simulink model "HVDCMMCInterconnection"  (R2023b)
settings: Solver=FixedStepDiscrete  StartTime=0.0  StopTime=10  FixedStep=Ts_Power  RelTol=1e-4
PreLoadFcn:
  | HVDCMMCInterconnectionParam
StartFcn:
  | tic
StopFcn:
  | toc
values from neighbouring files (symbols this model uses):
  C_PM = 1.758e-3    (= 0.001758)    [HVDCMMCInterconnectionParam.m]
  Cg = 50e-9    (= 5e-08)    [HVDCMMCInterconnectionParam.m]
  D_R = 0.001    [HVDCMMCInterconnectionParam.m]
  D_Rs = 1e8    (= 100000000)    [HVDCMMCInterconnectionParam.m]
  D_Vf = 0    [HVDCMMCInterconnectionParam.m]
  Fnom = 50    [HVDCMMCInterconnectionParam.m]
  HRM = 2    [HVDCMMCInterconnectionParam.m]
  Ki_Ireg = 6    [HVDCMMCInterconnectionParam.m]
  Ki_Preg = 1.0    (= 1)    [HVDCMMCInterconnectionParam.m]
  Ki_Qreg = 1.0    (= 1)    [HVDCMMCInterconnectionParam.m]
  Ki_VDCreg = 100    [HVDCMMCInterconnectionParam.m]
  Kp_Ireg = 0.6    [HVDCMMCInterconnectionParam.m]
  Kp_Preg = 0.5/3    (= 0.166666666667)    [HVDCMMCInterconnectionParam.m]
  Kp_Qreg = 0.5/3    (= 0.166666666667)    [HVDCMMCInterconnectionParam.m]
  Kp_VDCreg = 4    [HVDCMMCInterconnectionParam.m]
  L_cable = 15e-3    (= 0.015)    [HVDCMMCInterconnectionParam.m]
  Larm = Larm_pu*(Zb_ac/(2*pi*Fnom))    [HVDCMMCInterconnectionParam.m]
  Lff = Larm_pu/2    (= 0.075)    [HVDCMMCInterconnectionParam.m]
  Limits_Ireg = [ 2.0  -2.0]    [HVDCMMCInterconnectionParam.m]
  Limits_Preg = [ 1.2, 0.8 ]    [HVDCMMCInterconnectionParam.m]
  Limits_Qreg = [ 0.25, -0.25 ]    [HVDCMMCInterconnectionParam.m]
  Limits_VDCreg = [ 2.0  -2.0]    [HVDCMMCInterconnectionParam.m]
  Lxfo = 0.12    [HVDCMMCInterconnectionParam.m]
  Nb_PM = 36    [HVDCMMCInterconnectionParam.m]
  Pnom = 1000e6    (= 1000000000)    [HVDCMMCInterconnectionParam.m]
  R_cable = 0.5    [HVDCMMCInterconnectionParam.m]
  R_startup = 400    [HVDCMMCInterconnectionParam.m]
  Rarm = Rarm_pu*Zb_ac    [HVDCMMCInterconnectionParam.m]
  Rff = Rarm_pu/2    (= 0.00075)    [HVDCMMCInterconnectionParam.m]
  Rg = 100    [HVDCMMCInterconnectionParam.m]
  Rxfo = 0.003    [HVDCMMCInterconnectionParam.m]
  Slope_Pref = 0.5    [HVDCMMCInterconnectionParam.m]
  Slope_Qref = 0.5    [HVDCMMCInterconnectionParam.m]
  Slope_Vdc_ref = Vnom_dc/5    (= 128000)    [HVDCMMCInterconnectionParam.m]
  Tbrk1_On = 0.1    [HVDCMMCInterconnectionParam.m]
  Tbrk2_On = 1.0    (= 1)    [HVDCMMCInterconnectionParam.m]
  Tdeblock = 1.5    [HVDCMMCInterconnectionParam.m]
  Tfault = 9999    [HVDCMMCInterconnectionParam.m]
  Ton_Converter2 = 4    [HVDCMMCInterconnectionParam.m]
  Ton_PQreg = 4    [HVDCMMCInterconnectionParam.m]
  Ton_VDCreg = 1.5    [HVDCMMCInterconnectionParam.m]
  Ts = Ts_Control    (= 4e-05)    [HVDCMMCInterconnectionParam.m]    (also in power_circ2ss_sps_calc.m = 1e-06)
  Ts_Control = 40e-6    (= 4e-05)    [HVDCMMCInterconnectionParam.m]
  Ts_Power = 20e-6    (= 2e-05)    [HVDCMMCInterconnectionParam.m]
  Vb_ac = sqrt(2/3)*Vnom_sec    [HVDCMMCInterconnectionParam.m]
  Vb_dc = Vnom_dc    (= 640000)    [HVDCMMCInterconnectionParam.m]
  Vc0_PM = 0    [HVDCMMCInterconnectionParam.m]
  Vnom_dc = 640e3    (= 640000)    [HVDCMMCInterconnectionParam.m]
  Vnom_prim = 400e3    (= 400000)    [HVDCMMCInterconnectionParam.m]
  Vnom_sec = 333e3    (= 333000)    [HVDCMMCInterconnectionParam.m]
  w = 2*pi*Fnom    (= 314.159265359)    [HVDCMMCInterconnectionParam.m]
undefined symbols (not defined in the file or in its folder): ACDC, ACDC3, DiscIntNeverNeededParam, gcbh, Pcc, S, sps_AC, sps_rtmsupport
libraries: simulink x61, spsControlledVoltageSourceLib x56, spsCurrentMeasurementLib x56, spsDiodeLib x40, spsSeriesRLCBranchLib x32, spsVoltageMeasurementLib x20, powerlib_extras x9, spsHalfBridgeMMCmodel x8, spsGroundLib x7, spsSecondOrderFilterLib x6, spsabctodq0Lib x6, spsMeanLib x3
(part 3 of 11)

== system HVDCMMCInterconnection/Conv 2 ==
  On : Inport
  Add : Sum
  Bus Selector : BusSelector  OutputSignals=Switch current
  Bus Selector1 : BusSelector  OutputSignals=Switch current
  Constant2 : Constant  Value=Vnom_dc/2  SampleTime=Ts_Power
  Conv2SWn : spsIdealSwitchLib/Ideal Switch  Ron=0.001  Lon=0  IC=0  Rs=1e6  Cs=inf  Measurements=on
  Conv2SWp : spsIdealSwitchLib/Ideal Switch  Ron=0.001  Lon=0  IC=0  Rs=1e6  Cs=inf  Measurements=on
  Conv2VSn : spsControlledVoltageSourceLib/Controlled Voltage Source  Initialize=off  Source_Type=AC  Amplitude=0  Phase=0  Frequency=0  Measurements=None
  Conv2VSp : spsControlledVoltageSourceLib/Controlled Voltage Source  Initialize=off  Source_Type=AC  Amplitude=0  Phase=0  Frequency=0  Measurements=None
  Current Measurement1 : spsCurrentMeasurementLib/Current Measurement  PhasorSimulation=off  OutputType=Complex  PSBequivalent=0
  Current Measurement2 : spsCurrentMeasurementLib/Current Measurement  PhasorSimulation=off  OutputType=Complex  PSBequivalent=0
  Gain : Gain  Gain=0.5
  Gain1 : Gain  Gain=-1
  Ground1 : spsGroundLib/Ground  LConnTagsString=a
  Ground2 : spsGroundLib/Ground  LConnTagsString=a
  Voltage Measurement : spsVoltageMeasurementLib/Voltage Measurement  PhasorSimulation=off  OutputType=Complex  PSBequivalent=0
  Voltage Measurement1 : spsVoltageMeasurementLib/Voltage Measurement  PhasorSimulation=off  OutputType=Complex  PSBequivalent=0
  Voltage Measurement2 : spsVoltageMeasurementLib/Voltage Measurement  PhasorSimulation=off  OutputType=Complex  PSBequivalent=0
  + : PMIOPort  Side=Left
  -- : PMIOPort  Port=2  Side=Left
  tag scope: I_Conv2SWn=global, I_Conv2SWp=global, Idc2=global, Vdc2=global, Vdc2b=global, Vdc2t=global
  wires:
  On/1 -> Conv2SWn/1, Conv2SWp/1
  Current Measurement1/1 -> Add/1
  Current Measurement2/1 -> Gain1/1
  Add/1 -> Gain/1
  Gain/1 -> [Idc2]
  Gain1/1 -> Add/2
  Constant2/1 -> Conv2VSp/1, Conv2VSn/1
  Voltage Measurement/1 -> [Vdc2]
  Voltage Measurement1/1 -> [Vdc2t]
  Voltage Measurement2/1 -> [Vdc2b]
  Conv2SWp/1 -> Bus Selector/1
  Bus Selector/1 -> [I_Conv2SWp]  "<Switch current>"
  Conv2SWn/1 -> Bus Selector1/1
  Bus Selector1/1 -> [I_Conv2SWn]  "<Switch current>"
  connections:
  Conv2SWp/LConn1 -- Current Measurement1/RConn1
  Conv2VSn/LConn1 -- Conv2SWn/RConn1
  Conv2SWp/RConn1 -- Conv2VSp/RConn1
  Conv2VSn/RConn1 -- Conv2VSp/LConn1 -- Ground1/LConn1
  Current Measurement1/LConn1 -- Voltage Measurement/LConn1 -- +/RConn1 -- Voltage Measurement1/LConn1
  --/RConn1 -- Current Measurement2/LConn1 -- Voltage Measurement/LConn2 -- Voltage Measurement2/LConn2
  Current Measurement2/RConn1 -- Conv2SWn/LConn1
  Voltage Measurement1/LConn2 -- Voltage Measurement2/LConn1 -- Ground2/LConn1

== system HVDCMMCInterconnection/DC & converter 2 ==
  Add : Sum
  Cinv : spsSeriesRLCBranchLib/Series RLC Branch  LConnTagsString=__new0  RConnTagsString=__new0  BranchType=RC  Resistance=1e-3  Inductance=1e-3  SetiL0=off  InitialCurrent=0  Capacitance=C_PM/Nb_PM*3  Setx0=off  InitialVoltage=Vnom_dc/2  Measurements=None
  Cinv1 : spsSeriesRLCBranchLib/Series RLC Branch  LConnTagsString=__new0  RConnTagsString=__new0  BranchType=RC  Resistance=1e-3  Inductance=1e-3  SetiL0=off  InitialCurrent=0  Capacitance=C_PM/Nb_PM*3  Setx0=off  InitialVoltage=Vnom_dc/2  Measurements=None
  CnDC : spsSeriesRLCBranchLib/Series RLC Branch  LConnTagsString=__new0  RConnTagsString=__new0  BranchType=RC  Resistance=Rg  Inductance=1e-3  SetiL0=off  InitialCurrent=0  Capacitance=Cg  Setx0=off  InitialVoltage=Vnom_dc/2  Measurements=None
  CpDC : spsSeriesRLCBranchLib/Series RLC Branch  LConnTagsString=__new0  RConnTagsString=__new0  BranchType=RC  Resistance=Rg  Inductance=1e-3  SetiL0=off  InitialCurrent=0  Capacitance=Cg  Setx0=off  InitialVoltage=Vnom_dc/2  Measurements=None
  Gain : Gain  Gain=-0.5
  Gain1 : Gain  Gain=-1
  Ground2 : spsGroundLib/Ground  LConnTagsString=a
  Ground4 : spsGroundLib/Ground  LConnTagsString=a
  Idc1n : spsCurrentMeasurementLib/Current Measurement  PhasorSimulation=off  OutputType=Complex  PSBequivalent=0
  Idc1p : spsCurrentMeasurementLib/Current Measurement  PhasorSimulation=off  OutputType=Complex  PSBequivalent=0
  Vdc1 : spsVoltageMeasurementLib/Voltage Measurement  PhasorSimulation=off  OutputType=Complex  PSBequivalent=0
  Zcable1_1 : spsSeriesRLCBranchLib/Series RLC Branch  LConnTagsString=__new0  RConnTagsString=__new0  BranchType=RL  Resistance=R_cable  Inductance=L_cable  SetiL0=off  InitialCurrent=0  Capacitance=1e-6  Setx0=off  InitialVoltage=0  Measurements=None
  Zcable2_1 : spsSeriesRLCBranchLib/Series RLC Branch  LConnTagsString=__new0  RConnTagsString=__new0  BranchType=RL  Resistance=R_cable  Inductance=L_cable  SetiL0=off  InitialCurrent=0  Capacitance=1e-6  Setx0=off  InitialVoltage=0  Measurements=None
  Zcable5 : spsSeriesRLCBranchLib/Series RLC Branch  LConnTagsString=__new0  RConnTagsString=__new0  BranchType=RL  Resistance=1e-2+1e-3  Inductance=1e-4  SetiL0=off  InitialCurrent=0  Capacitance=1e-6  Setx0=off  InitialVoltage=0  Measurements=None
  Zcable6 : spsSeriesRLCBranchLib/Series RLC Branch  LConnTagsString=__new0  RConnTagsString=__new0  BranchType=RL  Resistance=1e-2+1e-3  Inductance=1e-4  SetiL0=off  InitialCurrent=0  Capacitance=1e-6  Setx0=off  InitialVoltage=0  Measurements=None
  1 : PMIOPort  Side=Left
  2 : PMIOPort  Port=2  Side=Left
  3 : PMIOPort  Port=3  Side=Right
  4 : PMIOPort  Port=4  Side=Right
  tag scope: Idc1=global, Vdc1=global
  wires:
  Vdc1/1 -> [Vdc1]
  Idc1p/1 -> Add/1
  Idc1n/1 -> Gain1/1
  Add/1 -> Gain/1
  Gain/1 -> [Idc1]
  Gain1/1 -> Add/2
  connections:
  Cinv1/LConn1 -- Ground2/LConn1 -- Cinv/RConn1
  Ground4/LConn1 -- CnDC/LConn1 -- CpDC/RConn1
  Zcable2_1/RConn1 -- Vdc1/LConn2 -- Idc1n/RConn1 -- CnDC/RConn1
  Zcable1_1/RConn1 -- Vdc1/LConn1 -- Idc1p/RConn1 -- CpDC/LConn1
  1/RConn1 -- Idc1p/LConn1
  Zcable6/RConn1 -- Zcable2_1/LConn1 -- Cinv1/RConn1
  Zcable5/LConn1 -- Zcable1_1/LConn1 -- Cinv/LConn1
  Idc1n/LConn1 -- 2/RConn1
  3/RConn1 -- Zcable5/RConn1
  4/RConn1 -- Zcable6/LConn1

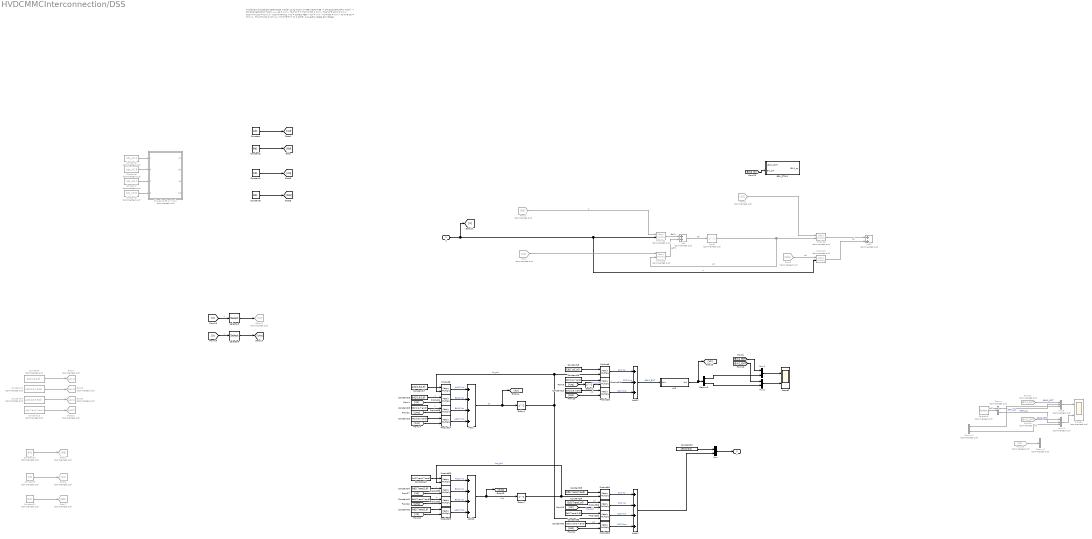
== system HVDCMMCInterconnection/DSS ==
  note: Implement discretized state-space model using Tustin or TBE method
      |
      | BE      -> SM.DSSmethod=1
      | Tustin  -> SM.DSSmethod=2
      |
      |
      | Tustin
      | ------
      | Ad = inv(I - Ts/2*A)*(I + Ts/2*A)
      | Bd = inv(I - Ts/2*A)*B
      | Cd = C*inv(I - Ts/2*A)*Ts
      | Dd = C*inv(I - Ts/2*A)*B*Ts/2  + D  =  Cd*B/2
      |
      | TBE
      | ---
      | Ad = inv(I - Ts*A)
      | Bd = inv(I - Ts*A)*B
      | Cd = C*inv(I - Ts*A)*Ts
      | Dd = C*inv(I - Ts*A)*B*Ts  + D  =  Cd*B
      |
      | I = eye(SM.nState,SM.nState)
  U : Inport
  Add : Sum  Commented=on
  Add1 : Sum  Inputs=++++
  Add10 : Sum  Inputs=++++
  Add11 : Sum  Inputs=++++
  Add12 : Sum  Inputs=+++
  Add2 : Sum  Commented=on
  BRK_CTRL1 : Subsystem
  Constant : Constant  Value=Ad1
  Constant1 : Constant  Value=Cd1
  Constant10 : Constant  Commented=on  Value=Bd1
  Constant11 : Constant  Commented=on  Value=Dd1
  Constant12 : Constant  Commented=on  Value=Ad1(1:6,7:end)
  Constant13 : Constant  Commented=on  Value=Ad1(7:end,7:end)
  Constant14 : Constant  Commented=on  Value=Ad1(1:6,7:end)
  Constant15 : Constant  Value=Ad1(1:6,7:end)
  Constant16 : Constant  Value=Cd1(1:6,7:end)
  Constant17 : Constant  Value=Ad1(1:6,1:6)
  Constant18 : Constant  Value=Bd1(1:6,1:6)
  Constant19 : Constant  Value=Cd1(1:6,1:6)
  Constant2 : Constant  Value=Bd1
  Constant20 : Constant  Value=zeros(6,1)
  Constant23 : Constant  Value=Dd1(1:6,7:end)
  Constant28 : Constant  Value=Bd1(1:6,7:end)
  Constant3 : Constant  Value=Dd1
  Constant35 : Constant  Value=Cd1(7:end,1:6)
  Constant37 : Constant  Value=Bd1(7:end,1:6)
  Constant38 : Constant  Value=Cd1(7:end,7:end)
  Constant39 : Constant  Value=Dd1(7:end,1:6)
  Constant4 : Constant  Commented=on  Value=Ad1(1:6,1:6)
  Constant40 : Constant  Value=Dd1(7:end,7:end)
  Constant41 : Constant  Value=Bd1(7:end,7:end)
  Constant42 : Constant  Value=Ad1(7:end,1:6)
  Constant43 : Constant  Value=Ad1(7:end,7:end)
  Constant5 : Constant  Commented=on  Value=sps_AC.A
  Constant6 : Constant  Commented=on  Value=sps_AC.B
  Constant7 : Constant  Commented=on  Value=sps_AC.C
  Constant8 : Constant  Commented=on  Value=sps_AC.D
  Constant9 : Constant  Commented=on  Value=Cd1
  Delay : Delay  Commented=on  DelayLength=1  InitialCondition=InitVec  SampleTime=dt
  Delay1 : Delay  DelayLength=1  InitialCondition=InitVec(1:6)  SampleTime=dt
  Delay2 : Delay  DelayLength=1  InitialCondition=InitVec(7:end)  SampleTime=dt
  Delay7 : Delay  DelayLength=1  InitialCondition=InitVec(7:end)  SampleTime=dt
  Demux : Demux  Commented=on  Outputs=2
  Demux1 : Demux  Commented=on  Outputs=2
  Demux2 : Demux  Commented=on  Outputs=2
  Demux3 : Demux  Outputs=2
  Discretize BE or Tustin : Subsystem  Commented=on  AncestorBlock="DQN_Machines/DQN_Mac_V1/Discretize  BE or Tustin"
  From : From  Commented=on  GotoTag=Ad
  From1 : From  Commented=on  GotoTag=Bd
  From2 : From  Commented=on  GotoTag=Cd
  From23 : From  Commented=on  GotoTag=Us
  From3 : From  Commented=on  GotoTag=Dd1
  From30 : From  Commented=on  GotoTag=UBrk2_EMT  TagVisibility=global
  From31 : From  Commented=on  GotoTag=UBrk1_EMT  TagVisibility=global
  Goto10 : Goto  Commented=on  GotoTag=Ad22
  Goto12 : Goto  Commented=on  GotoTag=Us
  Goto2 : Goto  Commented=on  GotoTag=Bd
  Goto4 : Goto  Commented=on  GotoTag=Ad11
  Goto6 : Goto  Commented=on  GotoTag=Cd
  Goto7 : Goto  Commented=on  GotoTag=Dd1
  Goto8 : Goto  Commented=on  GotoTag=Ad12
  Goto9 : Goto  Commented=on  GotoTag=Ad21
  Mux : Mux  Inputs=2
  Mux1 : Mux  Inputs=2
  Mux10 : Mux  Commented=on  Inputs=3
  Mux2 : Mux  Inputs=2
  Mux8 : Mux  Commented=on  Inputs=3
  Product{1..2,5,7} (4 alike) : Product  Commented=on  Multiplication=Matrix(*)  SaturateOnIntegerOverflow=on  OutDataTypeStr=Inherit: Same as first input
  Product{4,6,8,14..15,20,28..36} (15 alike) : Product  Multiplication=Matrix(*)  SaturateOnIntegerOverflow=on  OutDataTypeStr=Inherit: Same as first input
  Scope1 : Scope  Commented=on  NumInputPorts=2
  Scope2 : Scope  NumInputPorts=2
  Selector3 : Selector  Commented=on  InputPortWidth=33  IndexOptions=Index vector (dialog)  Indices=[1:6]  OutputSizes=1
  Selector5 : Selector  InputPortWidth=17  IndexOptions=Index vector (dialog)  Indices=[1:6]  OutputSizes=1
  Selector6 : Selector  InputPortWidth=17  IndexOptions=Index vector (dialog)  Indices=[7:17]  OutputSizes=1
  U-I2 : Subsystem
  Y : Outport
  wires:
  Constant/1 -> [Ad]
  Constant2/1 -> [Bd]
  Constant1/1 -> [Cd]
  Constant3/1 -> [Dd1]
  Constant7/1 -> Discretize BE or Tustin/3(C)
  Constant6/1 -> Discretize BE or Tustin/2(B)
  Constant8/1 -> Discretize BE or Tustin/4(D)
  Constant5/1 -> Discretize BE or Tustin/1(A)
  Product2/1 -> Add2/1
  U/1 -> Product7/2, Product1/2, [U]  "u"
  From1/1 -> Product1/1  "u"
  Delay/1 -> Product2/2, Product5/2  "xd"
  From3/1 -> Product7/1  "xd"
  Product1/1 -> Add/1  "Bd*U"
  Product7/1 -> Add2/2  "xd"
  Product5/1 -> Add/2  "Ad*X"
  From2/1 -> Product2/1
  From/1 -> Product5/1
  [Brk2_On] -> BRK_CTRL1/2(Brk_ON)
  ? -> BRK_CTRL1/1(UBrk1_EMT)  "UBrk2_EMT"
  Demux/2 -> Mux10/2  "IBrk2_ss"
  Mux10/1 -> Scope1/2
  From31/1 -> Mux8/1  "UBrk1_EMT"
  Mux8/1 -> Scope1/1
  From30/1 -> Mux10/1  "UBrk2_EMT"
  Demux/1 -> Mux8/2  "IBrk1_ss"
  Selector3/1 -> Demux/1  "Cd*Xnew"
  Constant4/1 -> Goto4/1
  Constant10/1 -> Goto2/1
  Constant9/1 -> Goto6/1
  Constant11/1 -> Goto7/1
  Constant12/1 -> Goto8/1
  Constant14/1 -> Goto9/1
  Constant13/1 -> Goto10/1
  Constant19/1 -> Product6/1
  Delay1/1 -> Product6/2, Product8/2, Product30/2  "Xs_old"
  Add1/1 -> [Xs], Delay1/1  "Xs"
  Constant18/1 -> Product4/1  "u"
  Constant17/1 -> Product8/1
  [Us] -> Product4/2
  [U] -> Selector5/1  "u"
  Selector5/1 -> Goto12/1
  [U] -> Selector6/1  "u"
  Selector6/1 -> [Uns]
  Demux1/1 -> Mux8/3
  Demux1/2 -> Mux10/3
  Constant15/1 -> Product14/1
  Product14/1 -> Add1/4  "Ad12*Xns"
  Constant16/1 -> Product15/1
  [Uns] -> Product20/2
  Constant23/1 -> Product20/1  "xd"
  Add/1 -> Delay/1  "xd"
  Delay7/1 -> Product35/2, Product34/2  "Xns_old"
  [Xns] -> Product14/2
  Product8/1 -> Add1/1  "Ad11*Xs"
  Product4/1 -> Add1/2  "Bd11*Us"
  Product28/1 -> Add1/3  "Bd11*Us"
  Constant28/1 -> Product28/1  "u"
  [Uns] -> Product28/2
  Product31/1 -> Add11/4  "D12*Uns"
  Product35/1 -> Add10/1  "Ad11*Xs"
  Constant40/1 -> Product31/1  "xd"
  Product30/1 -> Add11/3  "C12*Xns"
  Product32/1 -> Add10/3  "Bd11*Us"
  Product36/1 -> Add11/2  "D11*Us"
  Constant41/1 -> Product32/1  "u"
  Constant38/1 -> Product34/1
  Constant42/1 -> Product29/1
  Product34/1 -> Add11/1  "C11*Xs"
  Product33/1 -> Add10/2  "Bd11*Us"
  Constant43/1 -> Product35/1
  Constant37/1 -> Product33/1  "u"
  [Xs] -> Product29/2
  [Uns] -> Product32/2
  [Uns] -> Product31/2
  [Us] -> Product33/2
  Add10/1 -> [Xns], Delay7/1  "Xns"
  Constant35/1 -> Product30/1
  Constant39/1 -> Product36/1  "xd"
  Product29/1 -> Add10/4  "Ad12*Xns"
  From23/1 -> Demux2/1
  Product15/1 -> Add12/2  "C12*Xns"
  Product20/1 -> Add12/3  "D12*Uns"
  [IBrk2_EMT] -> Mux2/1
  Mux2/1 -> Scope2/2
  Mux1/1 -> Scope2/1
  [IBrk1_EMT] -> Mux1/1
  U-I2/1(Ibrk) -> [Us], Demux3/1
  Demux3/2 -> Mux2/2
  Demux3/1 -> Mux1/2
  Add11/1 -> Mux/2
  Mux/1 -> Y/1
  Product6/1 -> Add12/1  "C11*Xs"
  Add12/1 -> U-I2/1(Ubrk)  "UBrk1_EMT"
  Constant20/1 -> Mux/1
  [Xns] -> Delay2/1
  Delay2/1 -> Product15/2  "Xns_old"
  [Us] -> Product36/2  "Xns_old"

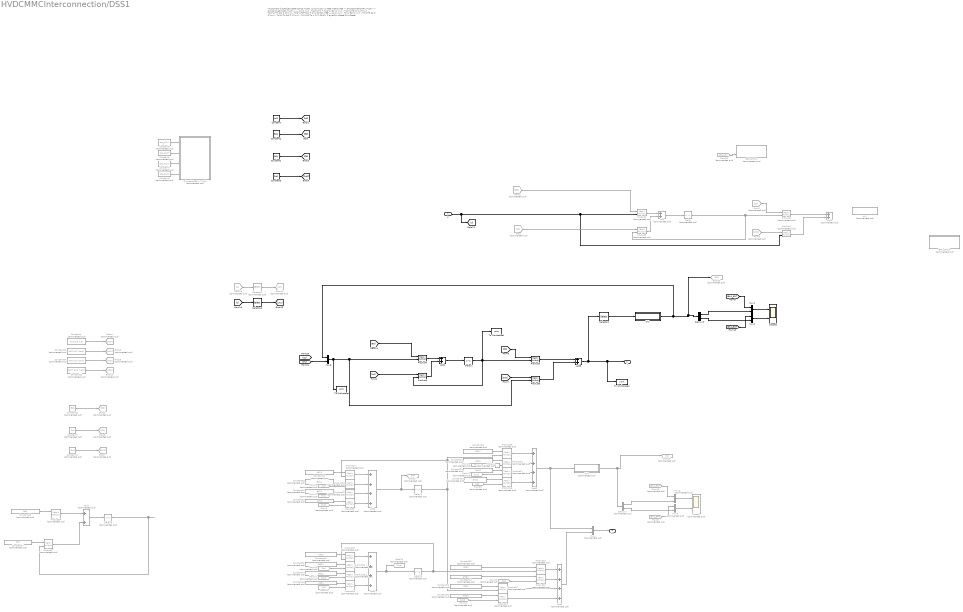
== system HVDCMMCInterconnection/DSS1 ==
  note: Implement discretized state-space model using Tustin or TBE method
      |
      | BE      -> SM.DSSmethod=1
      | Tustin  -> SM.DSSmethod=2
      |
      |
      | Tustin
      | ------
      | Ad = inv(I - Ts/2*A)*(I + Ts/2*A)
      | Bd = inv(I - Ts/2*A)*B
      | Cd = C*inv(I - Ts/2*A)*Ts
      | Dd = C*inv(I - Ts/2*A)*B*Ts/2  + D  =  Cd*B/2
      |
      | TBE
      | ---
      | Ad = inv(I - Ts*A)
      | Bd = inv(I - Ts*A)*B
      | Cd = C*inv(I - Ts*A)*Ts
      | Dd = C*inv(I - Ts*A)*B*Ts  + D  =  Cd*B
      |
      | I = eye(SM.nState,SM.nState)
  U : Inport
  Add : Sum  Commented=on
  Add1 : Sum
  Add2 : Sum  Commented=on
  Add{3..6} (4 alike) : Sum  Commented=on  Inputs=++++
  Add7 : Sum  Commented=on
  Add8 : Sum
  BRK_CTRL1 : Subsystem  Commented=on
  BRK_CTRL3 : Subsystem  Commented=on
  Constant : Constant  Value=Ad1
  Constant1 : Constant  Value=Cd1
  Constant10 : Constant  Commented=on  Value=Bd1
  Constant11 : Constant  Commented=on  Value=Dd1
  Constant12 : Constant  Commented=on  Value=Ad1(1:6,7:end)
  Constant13 : Constant  Commented=on  Value=Ad1(7:end,7:end)
  Constant14 : Constant  Commented=on  Value=Ad1(1:6,7:end)
  Constant2 : Constant  Value=Bd1
  Constant20 : Constant  Commented=on  Value=Ad12
  Constant22 : Constant  Commented=on  Value=Cd12
  Constant24 : Constant  Commented=on  Value=Ad11
  Constant25 : Constant  Commented=on  Value=Bd11
  Constant26 : Constant  Commented=on  Value=Cd11
  Constant27 : Constant  Commented=on  Value=Dd11
  Constant29 : Constant  Commented=on  Value=Dd12
  Constant3 : Constant  Value=Dd1
  Constant30 : Constant  Commented=on  Value=Bd12
  Constant31 : Constant  Commented=on  Value=Cd21
  Constant32 : Constant  Commented=on  Value=Bd21
  Constant33 : Constant  Commented=on  Value=Cd22
  Constant34 : Constant  Commented=on  Value=Dd21
  Constant36 : Constant  Commented=on  Value=Dd22
  Constant4 : Constant  Commented=on  Value=Ad1(1:6,1:6)
  Constant44 : Constant  Commented=on  Value=Bd22
  Constant45 : Constant  Commented=on  Value=Ad21
  Constant46 : Constant  Commented=on  Value=Ad22
  Constant47 : Constant  Commented=on  Value=Ad1
  Constant48 : Constant  Commented=on  Value=Bd1
  Constant5 : Constant  Commented=on  Value=sps_AC.A
  Constant6 : Constant  Commented=on  Value=sps_AC.B
  Constant7 : Constant  Commented=on  Value=sps_AC.C
  Constant8 : Constant  Commented=on  Value=sps_AC.D
  Constant9 : Constant  Commented=on  Value=Cd1
  Delay : Delay  Commented=on  DelayLength=1  InitialCondition=InitVec  SampleTime=dt
  Delay1 : Delay  DelayLength=1  InitialCondition=InitVec  SampleTime=dt
  Delay3 : Delay  Commented=on  DelayLength=1  InitialCondition=InitVecS  SampleTime=dt
  Delay4 : Delay  Commented=on  DelayLength=1  InitialCondition=InitVecNS  SampleTime=dt
  Delay5 : Delay  Commented=on  DelayLength=1  InitialCondition=InitVecNS  SampleTime=dt
  Delay6 : Delay  Commented=on  DelayLength=1  InitialCondition=InitVec  SampleTime=dt
  Demux1 : Demux  Commented=on  Outputs=2
  Demux3 : Demux  Outputs=2
  Discretize BE or Tustin : Subsystem  Commented=on  AncestorBlock="DQN_Machines/DQN_Mac_V1/Discretize  BE or Tustin"
  From : From  Commented=on  GotoTag=Ad
  From1 : From  Commented=on  GotoTag=Bd
  From{11..13,17} (4 alike) : From  Commented=on  GotoTag=Uns
  From15 : From  Commented=on  GotoTag=U
  From{18,20,23,30} (4 alike) : From  Commented=on  GotoTag=Us
  From19 : From  Commented=on  GotoTag=IBrk1_EMT  TagVisibility=global
  From2 : From  Commented=on  GotoTag=Cd
  From22 : From  Commented=on  GotoTag=Xs
  From25 : From  Commented=on  GotoTag=Xns
  From29 : From  Commented=on  GotoTag=Brk2_On  TagVisibility=global
  From3 : From  Commented=on  GotoTag=Dd1
  From6 : From  Commented=on  GotoTag=Xns
  From9 : From  Commented=on  GotoTag=IBrk2_EMT  TagVisibility=global
  Goto10 : Goto  Commented=on  GotoTag=Ad22
  Goto12 : Goto  Commented=on  GotoTag=Us
  Goto15 : Goto  Commented=on  GotoTag=Us
  Goto17 : Goto  Commented=on  GotoTag=Xs
  Goto18 : Goto  Commented=on  GotoTag=Us
  Goto19 : Goto  Commented=on  GotoTag=Xns
  Goto2 : Goto  Commented=on  GotoTag=Bd
  Goto4 : Goto  Commented=on  GotoTag=Ad11
  Goto6 : Goto  Commented=on  GotoTag=Cd
  Goto7 : Goto  Commented=on  GotoTag=Dd1
  Goto8 : Goto  Commented=on  GotoTag=Ad12
  Goto9 : Goto  Commented=on  GotoTag=Ad21
  Mux1 : Mux  Inputs=2
  Mux2 : Mux  Inputs=2
  Mux3 : Mux  Commented=on  Inputs=2
  Mux4 : Mux  Commented=on  Inputs=2
  Mux5 : Mux  Commented=on  Inputs=2
  Mux6 : Mux  Inputs=2
  Product{1..2,5,7,9..13,16..19,21..27,37..38} (22 alike) : Product  Commented=on  Multiplication=Matrix(*)  SaturateOnIntegerOverflow=on  OutDataTypeStr=Inherit: Same as first input
  Product{3..4,6,8} (4 alike) : Product  Multiplication=Matrix(*)  SaturateOnIntegerOverflow=on  OutDataTypeStr=Inherit: Same as first input
  Scope1 : Scope  Commented=on  NumInputPorts=2
  Scope2 : Scope  NumInputPorts=2
  Selector1 : Selector  InputPortWidth=size(Cd1,1)  IndexOptions=Index vector (dialog)  Indices=[1:NrBrk]  OutputSizes=1
  Selector2 : Selector  Commented=on  InputPortWidth=size(B,2)  IndexOptions=Index vector (dialog)  Indices=[1:NrBrk]  OutputSizes=1
  Selector6 : Selector  InputPortWidth=size(B,2)  IndexOptions=Index vector (dialog)  Indices=[NrBrk+1:size(B,2)]  OutputSizes=1
  To Workspace : ToWorkspace  VariableName=usim  SampleTime=Ts_Power
      settings: Save2DSignal=2-D array (concatenate along first dimension)
  To Workspace1 : ToWorkspace  VariableName=xsim  SampleTime=Ts_Power
      settings: Save2DSignal=2-D array (concatenate along first dimension)
  To Workspace2 : ToWorkspace  VariableName=ysim  SampleTime=Ts_Power
      settings: Save2DSignal=2-D array (concatenate along first dimension)
  U-I1 : Subsystem
  U-I2 : Subsystem  Commented=on
  U-I3 : Subsystem  Commented=on
  Y : Outport
  Y1 : Outport  Port=2
  wires:
  Constant/1 -> [Ad]
  Constant2/1 -> [Bd]
  Constant1/1 -> [Cd]
  Constant3/1 -> [Dd1]
  Constant7/1 -> Discretize BE or Tustin/3(C)
  Constant6/1 -> Discretize BE or Tustin/2(B)
  Constant8/1 -> Discretize BE or Tustin/4(D)
  Constant5/1 -> Discretize BE or Tustin/1(A)
  Product2/1 -> Add2/1
  U/1 -> [U], Product7/2, Product1/2  "u"
  From1/1 -> Product1/1  "u"
  Delay/1 -> Product2/2, Product5/2  "xd"
  From3/1 -> Product7/1  "xd"
  Product1/1 -> Add/1  "Bd*U"
  Product7/1 -> Add2/2  "xd"
  Product5/1 -> Add/2  "Ad*X"
  From2/1 -> Product2/1
  From/1 -> Product5/1
  From29/1 -> BRK_CTRL1/2(Brk_ON)
  ? -> BRK_CTRL1/1(UBrk1_EMT)  "UBrk2_EMT"
  Constant4/1 -> Goto4/1
  Constant10/1 -> Goto2/1
  Constant9/1 -> Goto6/1
  Constant11/1 -> Goto7/1
  Constant12/1 -> Goto8/1
  Constant14/1 -> Goto9/1
  Constant13/1 -> Goto10/1
  From15/1 -> Selector2/1  "u"
  Selector2/1 -> Goto12/1
  [U] -> Selector6/1  "u"
  Selector6/1 -> [Uns]
  Add/1 -> Delay/1  "xd"
  [IBrk2_EMT] -> Mux2/1
  Mux2/1 -> Scope2/2
  Mux1/1 -> Scope2/1
  [IBrk1_EMT] -> Mux1/1
  Demux3/2 -> Mux2/2
  Demux3/1 -> Mux1/2
  Product10/1 -> Add6/2  "C12*Xns"
  Constant45/1 -> Product13/1
  Add6/1 -> Mux4/1, U-I3/1(Ubrk)  "UBrk1_EMT"
  Product16/1 -> Add6/4  "D11*Us"
  Constant46/1 -> Product23/1
  From17/1 -> Product19/2
  U-I3/1(Ibrk) -> Demux1/1, Goto18/1
  Product24/1 -> Add5/2  "D11*Us"
  Constant27/1 -> Product16/1  "xd"
  From13/1 -> Product18/2
  Constant20/1 -> Product9/1
  Delay4/1 -> Product10/2  "Xns_old"
  Product19/1 -> Add4/3  "Bd22*Us"
  Constant25/1 -> Product25/1  "u"
  From23/1 -> Product25/2
  Constant34/1 -> Product24/1
  Product11/1 -> Add6/3  "D12*Uns"
  From25/1 -> Delay4/1
  Add5/1 -> Mux4/2
  Product21/1 -> Add4/2  "Bd21*Us"
  From18/1 -> Product21/2
  Constant29/1 -> Product11/1  "xd"
  Constant36/1 -> Product18/1  "xd"
  Constant22/1 -> Product10/1
  Constant33/1 -> Product22/1
  From22/1 -> Product13/2
  Product13/1 -> Add4/4  "Ad21*Xns"
  Add4/1 -> Goto19/1, Delay5/1  "Xns"
  Constant24/1 -> Product27/1
  Product22/1 -> Add5/1  "C11*Xs"
  Product26/1 -> Add6/1  "C11*Xs"
  Constant31/1 -> Product17/1
  Constant44/1 -> Product19/1  "u"
  Constant32/1 -> Product21/1  "u"
  Product17/1 -> Add5/3  "C12*Xns"
  Product9/1 -> Add3/4  "Ad12*Xns"
  Product12/1 -> Add3/3  "Bd12*Us"
  From30/1 -> Product16/2
  From11/1 -> Product11/2
  From6/1 -> Product9/2
  Product25/1 -> Add3/2  "Bd11*Us"
  From12/1 -> Product12/2
  Constant30/1 -> Product12/1  "u"
  Product27/1 -> Add3/1  "Ad11*Xs"
  Delay5/1 -> Product22/2, Product23/2
  Delay3/1 -> Product26/2, Product27/2, Product17/2  "Xs_old"
  Product18/1 -> Add5/4  "D12*Uns"
  Add3/1 -> Goto17/1, Delay3/1  "Xs"
  Product23/1 -> Add4/1  "Ad22*Xs"
  Constant26/1 -> Product26/1
  From20/1 -> Product24/2
  Mux4/1 -> Y1/1
  Add1/1 -> Delay1/1  "xd"
  [Ad] -> Product8/1
  Mux6/1 -> To Workspace/1, Product6/2, Product4/2  "u"
  Product8/1 -> Add1/2  "Ad*X"
  Product4/1 -> Add1/1  "Bd*U"
  [Bd] -> Product4/1  "u"
  [Uns] -> Mux6/2
  Delay6/1 -> Product37/2  "Xs_old"
  Product37/1 -> Add7/2  "Ad11*Xs"
  Constant47/1 -> Product37/1
  Add7/1 -> Delay6/1
  Product38/1 -> Add7/1  "Ad11*Xs"
  Constant48/1 -> Product38/1
  Delay1/1 -> To Workspace1/1, Product8/2, Product3/2  "xd"
  Product6/1 -> Add8/2  "xd"
  [Cd] -> Product3/1
  [Dd1] -> Product6/1  "xd"
  Product3/1 -> Add8/1
  Add8/1 -> Selector1/1, To Workspace2/1, Y/1
  Selector1/1 -> U-I1/1(Ubrk)  "Ys"
  U-I1/1(Ibrk) -> Mux6/1, Goto15/1, Demux3/1  "Us"
  From19/1 -> Mux3/1
  From9/1 -> Mux5/1
  Mux5/1 -> Scope1/2
  Mux3/1 -> Scope1/1
  Demux1/2 -> Mux5/2
  Demux1/1 -> Mux3/2

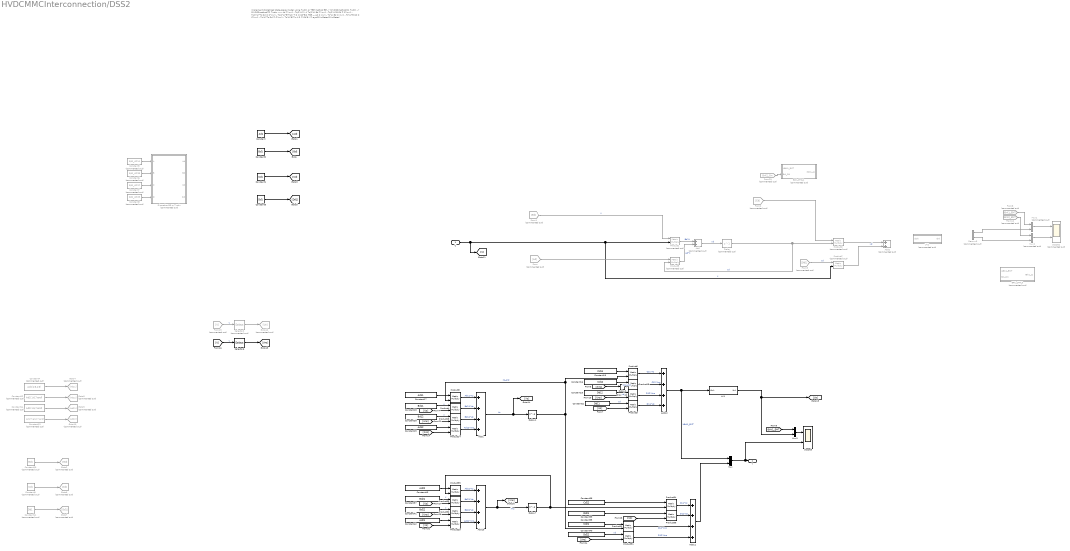
== system HVDCMMCInterconnection/DSS2 ==
  note: Implement discretized state-space model using Tustin or TBE method
      |
      | BE      -> SM.DSSmethod=1
      | Tustin  -> SM.DSSmethod=2
      |
      |
      | Tustin
      | ------
      | Ad = inv(I - Ts/2*A)*(I + Ts/2*A)
      | Bd = inv(I - Ts/2*A)*B
      | Cd = C*inv(I - Ts/2*A)*Ts
      | Dd = C*inv(I - Ts/2*A)*B*Ts/2  + D  =  Cd*B/2
      |
      | TBE
      | ---
      | Ad = inv(I - Ts*A)
      | Bd = inv(I - Ts*A)*B
      | Cd = C*inv(I - Ts*A)*Ts
      | Dd = C*inv(I - Ts*A)*B*Ts  + D  =  Cd*B
      |
      | I = eye(SM.nState,SM.nState)
  U : Inport
  Add : Sum  Commented=on
  Add{1,10..12} (4 alike) : Sum  Inputs=++++
  Add2 : Sum  Commented=on
  BRK_CTRL1 : Subsystem  Commented=on
  BRK_CTRL3 : Subsystem  Commented=on
  Constant : Constant  Value=Ad1
  Constant1 : Constant  Value=Cd1
  Constant10 : Constant  Commented=on  Value=Bd1
  Constant11 : Constant  Commented=on  Value=Dd1
  Constant12 : Constant  Commented=on  Value=Ad1(1:6,7:end)
  Constant13 : Constant  Commented=on  Value=Ad1(7:end,7:end)
  Constant14 : Constant  Commented=on  Value=Ad1(1:6,7:end)
  Constant15 : Constant  Value=Ad12
  Constant16 : Constant  Value=Cd12
  Constant17 : Constant  Value=Ad11
  Constant18 : Constant  Value=Bd11
  Constant19 : Constant  Value=Cd11
  Constant2 : Constant  Value=Bd1
  Constant21 : Constant  Value=Dd11
  Constant23 : Constant  Value=Dd12
  Constant28 : Constant  Value=Bd12
  Constant3 : Constant  Value=Dd1
  Constant35 : Constant  Value=Cd21
  Constant37 : Constant  Value=Bd21
  Constant38 : Constant  Value=Cd22
  Constant39 : Constant  Value=Dd21
  Constant4 : Constant  Commented=on  Value=Ad1(1:6,1:6)
  Constant40 : Constant  Value=Dd22
  Constant41 : Constant  Value=Bd22
  Constant42 : Constant  Value=Ad21
  Constant43 : Constant  Value=Ad22
  Constant5 : Constant  Commented=on  Value=sps_AC.A
  Constant6 : Constant  Commented=on  Value=sps_AC.B
  Constant7 : Constant  Commented=on  Value=sps_AC.C
  Constant8 : Constant  Commented=on  Value=sps_AC.D
  Constant9 : Constant  Commented=on  Value=Cd1
  Delay : Delay  Commented=on  DelayLength=1  InitialCondition=InitVec  SampleTime=dt
  Delay1 : Delay  DelayLength=1  InitialCondition=InitVecS  SampleTime=dt
  Delay2 : Delay  DelayLength=1  InitialCondition=InitVecNS  SampleTime=dt
  Delay7 : Delay  DelayLength=1  InitialCondition=InitVecNS  SampleTime=dt
  Demux3 : Demux  Commented=on  Outputs=2
  Discretize BE or Tustin : Subsystem  Commented=on  AncestorBlock="DQN_Machines/DQN_Mac_V1/Discretize  BE or Tustin"
  From : From  Commented=on  GotoTag=Ad
  From1 : From  Commented=on  GotoTag=Bd
  From10 : From  Commented=on  GotoTag=IBrk2_EMT  TagVisibility=global
  From15 : From  Commented=on  GotoTag=U
  From2 : From  Commented=on  GotoTag=Cd
  From29 : From  Commented=on  GotoTag=Brk2_On  TagVisibility=global
  From3 : From  Commented=on  GotoTag=Dd1
  From8 : From  Commented=on  GotoTag=IBrk1_EMT  TagVisibility=global
  Goto10 : Goto  Commented=on  GotoTag=Ad22
  Goto12 : Goto  Commented=on  GotoTag=Us
  Goto2 : Goto  Commented=on  GotoTag=Bd
  Goto4 : Goto  Commented=on  GotoTag=Ad11
  Goto6 : Goto  Commented=on  GotoTag=Cd
  Goto7 : Goto  Commented=on  GotoTag=Dd1
  Goto8 : Goto  Commented=on  GotoTag=Ad12
  Goto9 : Goto  Commented=on  GotoTag=Ad21
  Mux : Mux  Inputs=2
  Mux1 : Mux  Commented=on  Inputs=2
  Mux2 : Mux  Commented=on  Inputs=2
  Mux3 : Mux  Inputs=2
  Product{1..2,5,7} (4 alike) : Product  Commented=on  Multiplication=Matrix(*)  SaturateOnIntegerOverflow=on  OutDataTypeStr=Inherit: Same as first input
  Product{3..4,6,8,14..15,20,28..36} (16 alike) : Product  Multiplication=Matrix(*)  SaturateOnIntegerOverflow=on  OutDataTypeStr=Inherit: Same as first input
  Scope2 : Scope  Commented=on  NumInputPorts=2
  Scope3 : Scope  NumInputPorts=2
  Selector2 : Selector  Commented=on  InputPortWidth=size(B,2)  IndexOptions=Index vector (dialog)  Indices=[1:NrBrk]  OutputSizes=1
  Selector6 : Selector  InputPortWidth=size(B,2)  IndexOptions=Index vector (dialog)  Indices=[NrBrk+1:size(B,2)]  OutputSizes=1
  U-I1 : Subsystem
  U-I2 : Subsystem  Commented=on
  Y : Outport
  wires:
  Constant/1 -> [Ad]
  Constant2/1 -> [Bd]
  Constant1/1 -> [Cd]
  Constant3/1 -> [Dd1]
  Constant7/1 -> Discretize BE or Tustin/3(C)
  Constant6/1 -> Discretize BE or Tustin/2(B)
  Constant8/1 -> Discretize BE or Tustin/4(D)
  Constant5/1 -> Discretize BE or Tustin/1(A)
  Product2/1 -> Add2/1
  U/1 -> [U], Product7/2, Product1/2  "u"
  From1/1 -> Product1/1  "u"
  Delay/1 -> Product2/2, Product5/2  "xd"
  From3/1 -> Product7/1  "xd"
  Product1/1 -> Add/1  "Bd*U"
  Product7/1 -> Add2/2  "xd"
  Product5/1 -> Add/2  "Ad*X"
  From2/1 -> Product2/1
  From/1 -> Product5/1
  From29/1 -> BRK_CTRL1/2(Brk_ON)
  ? -> BRK_CTRL1/1(UBrk1_EMT)  "UBrk2_EMT"
  Constant4/1 -> Goto4/1
  Constant10/1 -> Goto2/1
  Constant9/1 -> Goto6/1
  Constant11/1 -> Goto7/1
  Constant12/1 -> Goto8/1
  Constant14/1 -> Goto9/1
  Constant13/1 -> Goto10/1
  Constant19/1 -> Product6/1
  Delay1/1 -> Product6/2, Product8/2, Product30/2  "Xs_old"
  Add1/1 -> [Xs], Delay1/1  "Xs"
  Constant18/1 -> Product4/1  "u"
  Constant17/1 -> Product8/1
  [Us] -> Product4/2
  From15/1 -> Selector2/1  "u"
  Selector2/1 -> Goto12/1
  [U] -> Selector6/1  "u"
  Selector6/1 -> [Uns]
  Constant15/1 -> Product14/1
  Product14/1 -> Add1/4  "Ad12*Xns"
  Constant16/1 -> Product15/1
  [Uns] -> Product20/2
  Constant23/1 -> Product20/1  "xd"
  Add/1 -> Delay/1  "xd"
  Delay7/1 -> Product34/2, Product35/2
  [Xns] -> Product14/2
  Product8/1 -> Add1/1  "Ad11*Xs"
  Product4/1 -> Add1/2  "Bd11*Us"
  Product28/1 -> Add1/3  "Bd12*Us"
  Constant28/1 -> Product28/1  "u"
  [Uns] -> Product28/2
  Product31/1 -> Add11/4  "D12*Uns"
  Product35/1 -> Add10/1  "Ad22*Xs"
  Constant40/1 -> Product31/1  "xd"
  Product30/1 -> Add11/3  "C12*Xns"
  Product32/1 -> Add10/3  "Bd22*Us"
  Product36/1 -> Add11/2  "D11*Us"
  Constant41/1 -> Product32/1  "u"
  Constant38/1 -> Product34/1
  Constant42/1 -> Product29/1
  Product34/1 -> Add11/1  "C11*Xs"
  Product33/1 -> Add10/2  "Bd21*Us"
  Constant43/1 -> Product35/1
  Constant37/1 -> Product33/1  "u"
  [Xs] -> Product29/2
  [Uns] -> Product32/2
  [Uns] -> Product31/2
  [Us] -> Product33/2
  Add10/1 -> [Xns], Delay7/1  "Xns"
  Constant35/1 -> Product30/1
  Constant39/1 -> Product36/1
  Product29/1 -> Add10/4  "Ad21*Xns"
  Product15/1 -> Add12/2  "C12*Xns"
  Product20/1 -> Add12/3  "D12*Uns"
  From10/1 -> Mux2/1
  Mux2/1 -> Scope2/2
  Mux1/1 -> Scope2/1
  From8/1 -> Mux1/1
  ? -> Demux3/1
  Demux3/2 -> Mux2/2
  Demux3/1 -> Mux1/2
  Add11/1 -> Mux/2
  Mux/1 -> Scope3/2, Y/1
  Product6/1 -> Add12/1  "C11*Xs"
  [Xns] -> Delay2/1
  Delay2/1 -> Product15/2  "Xns_old"
  Constant21/1 -> Product3/1  "xd"
  [Us] -> Product3/2
  U-I1/1(Ibrk) -> Mux3/2, [Us]
  [Us] -> Product36/2
  Mux3/1 -> Scope3/1
  [IBrk1_EMT] -> Mux3/1
  Add12/1 -> Mux/1, U-I1/1(Ubrk)  "UBrk1_EMT"
  Product3/1 -> Add12/4  "D11*Us"

== system HVDCMMCInterconnection/Delay5 ==
  In1 : Inport
  Gain3 : Gain  Gain=0.5
  Sum4 : Sum  InputSameDT=on  SaturateOnIntegerOverflow=on  OutDataTypeStr=Inherit: Same as first input
  Unit Delay6 : UnitDelay  SampleTime=Ts_Power  HasFrameUpgradeWarning=on
  Out1 : Outport
  wires:
  In1/1 -> Sum4/2, Unit Delay6/1
  Unit Delay6/1 -> Sum4/1
  Sum4/1 -> Gain3/1
  Gain3/1 -> Out1/1

== system HVDCMMCInterconnection/Delay6 ==
  In1 : Inport
  Gain3 : Gain  Gain=0.5
  Sum4 : Sum  InputSameDT=on  SaturateOnIntegerOverflow=on  OutDataTypeStr=Inherit: Same as first input
  Unit Delay6 : UnitDelay  SampleTime=Ts_Power  HasFrameUpgradeWarning=on
  Out1 : Outport
  wires:
  In1/1 -> Sum4/2, Unit Delay6/1
  Unit Delay6/1 -> Sum4/1
  Sum4/1 -> Gain3/1
  Gain3/1 -> Out1/1

== system HVDCMMCInterconnection/Delay7 ==
  In1 : Inport
  Gain3 : Gain  Gain=0.5
  Sum4 : Sum  InputSameDT=on  SaturateOnIntegerOverflow=on  OutDataTypeStr=Inherit: Same as first input
  Unit Delay6 : UnitDelay  SampleTime=Ts_Power  HasFrameUpgradeWarning=on
  Out1 : Outport
  wires:
  In1/1 -> Sum4/2, Unit Delay6/1
  Unit Delay6/1 -> Sum4/1
  Sum4/1 -> Gain3/1
  Gain3/1 -> Out1/1

== system HVDCMMCInterconnection/Delay8 ==
  In1 : Inport
  Gain3 : Gain  Gain=0.5
  Sum4 : Sum  InputSameDT=on  SaturateOnIntegerOverflow=on  OutDataTypeStr=Inherit: Same as first input
  Unit Delay6 : UnitDelay  SampleTime=Ts_Power  HasFrameUpgradeWarning=on
  Out1 : Outport
  wires:
  In1/1 -> Sum4/2, Unit Delay6/1
  Unit Delay6/1 -> Sum4/1
  Sum4/1 -> Gain3/1
  Gain3/1 -> Out1/1

== system HVDCMMCInterconnection/Delay9 ==
  In1 : Inport
  Gain3 : Gain  Gain=0.5
  Sum4 : Sum  InputSameDT=on  SaturateOnIntegerOverflow=on  OutDataTypeStr=Inherit: Same as first input
  Unit Delay6 : UnitDelay  SampleTime=Ts_Power  HasFrameUpgradeWarning=on
  Out1 : Outport
  wires:
  In1/1 -> Sum4/2, Unit Delay6/1
  Unit Delay6/1 -> Sum4/1
  Sum4/1 -> Gain3/1
  Gain3/1 -> Out1/1

== system HVDCMMCInterconnection/Gates1 ==
  Mux : Mux  Inputs=[1 1 1 1 1 1 1 1 1 1 1 1 1 1 1 1 1 1 1 1]
  gates : Outport  VectorParamsAs1DForOutWhenUnconnected=off
  wires:
  Mux/1 -> gates/1
  [T43_3874_2886452653200] -> Mux/1
  [T43_3876_2899958850653] -> Mux/2
  [T42_3783_2668712860261] -> Mux/3
  [T42_3784_2670194316057] -> Mux/4
  [T42_3785_2671784573757] -> Mux/5
  [T42_3784_2667400997265] -> Mux/6
  [T42_3785_2668880521074] -> Mux/7
  [T42_3786_2670468846789] -> Mux/8
  [T41_3578_2337987065122] -> Mux/9
  [T41_3596_2447714498780] -> Mux/10
  [T41_3582_2355687534878] -> Mux/11
  [T41_3600_2465248997561] -> Mux/12
  [T41_3580_2338929198402] -> Mux/13
  [T41_3598_2448576300476] -> Mux/14
  [T41_3584_2356614062524] -> Mux/15
  [T41_3602_2466095193622] -> Mux/16
  [T41_3582_2340019000902] -> Mux/17
  [T41_3600_2449585771390] -> Mux/18
  [T41_3586_2357688259390] -> Mux/19
  [T41_3604_2467089058902] -> Mux/20
